simulink model "BodyQuarter_Verif"  (R2021b)
settings: Solver=VariableStepAuto  StartTime=0.0  StopTime=10.0  RelTol=1e-3
values from neighbouring files (symbols this model uses):
  M1 = 500    [CarQuarterParam.m]
settings Model: Creator=Reece Bell  LastModifiedBy=reece
settings SolverCC: AlgebraicLoopSolver=TrustRegion
settings DataIOCC: ReturnWorkspaceOutputs=off
settings DebuggingCC: SFMachineParentedDataDiag=warning  ArithmeticOperatorsInVariantConditions=warning
settings SFSimCC: CustomCodeUndefinedFunction=UseInterfaceOnly

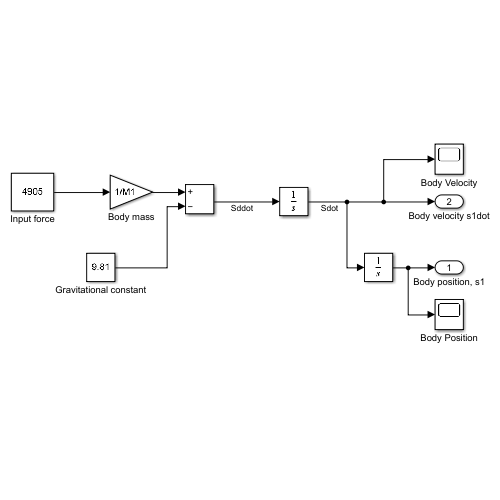
[thumbnail: Simulink's stored preview of the top-level diagram]
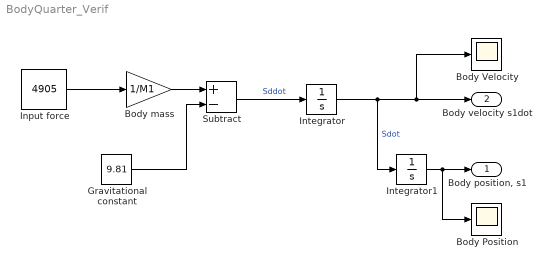
== system BodyQuarter_Verif ==
  "Body Position " : Scope
  "Body Velocity " : Scope
  "Body mass " : Gain  Gain=1/M1
  Gravitational constant : Constant  Value=9.81
  "Input force " : Constant  Value=4905
  Integrator : Integrator
  Integrator1 : Integrator
  Subtract : Sum  Inputs=+-
  "Body position, s1" : Outport  VectorParamsAs1DForOutWhenUnconnected=off
  "Body velocity s1dot " : Outport  Port=2  VectorParamsAs1DForOutWhenUnconnected=off
  wires:
  Integrator/1 -> Integrator1/1, "Body velocity s1dot "/1, "Body Velocity "/1  "Sdot"
  "Body mass "/1 -> Subtract/1
  Subtract/1 -> Integrator/1  "Sddot"
  "Input force "/1 -> "Body mass "/1
  Integrator1/1 -> "Body position, s1"/1, "Body Position "/1
  Gravitational constant/1 -> Subtract/2
